simulink model "sam"  (R2016b)
settings: Solver=VariableStepAuto  StartTime=0.0  StopTime=10  FixedStep=0.00001
values from neighbouring files (symbols this model uses):
  J = 0.0025    [momentFun.m]
  K = Kf*R/Km+Ke    (= 4.8)    [momentFun.m]
  Kd = Kn(3)    [momentFun.m]
  Ki = Kn(2)    [momentFun.m]
  Km = 4.8    [momentFun.m]
  Kp = Kn(1)    [momentFun.m]
  maxV = 6.8    [momentFun.m]
  R = 5.2    [momentFun.m]
libraries: simulink x1
settings Model: Creator=texnoman  LastModifiedBy=texnoman
settings SolverCC: MaxConsecutiveMinStep=auto  ZeroCrossControl=DisableAll

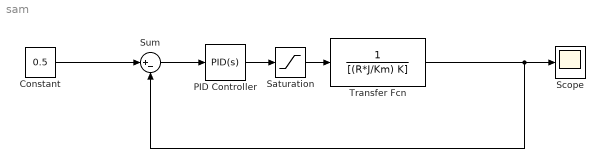
== system sam ==
  Constant : Constant  Value=0.5
  PID Controller : simulink/Continuous/PID Controller  Controller=PID  TimeDomain=Continuous-time  SampleTime=-1  IntegratorMethod=Forward Euler  FilterMethod=Forward Euler  Form=Parallel  UseFilter=on  ControllerParametersSource=internal  P=Kp  I=Ki  D=Kd  N=100  InitialConditionSource=internal  InitialConditionForIntegrator=0  InitialConditionForFilter=0  ExternalReset=none  LimitOutput=off  UpperSaturationLimit=inf  LowerSaturationLimit=-inf  LinearizeAsGain=on  AntiWindupMode=none  Kb=1  TrackingMode=off  Kt=1  PParamMin=[]  PParamMax=[]  IParamMin=[]  IParamMax=[]  DParamMin=[]  DParamMax=[]  NParamMin=[]  NParamMax=[]  KbParamMin=[]  KbParamMax=[]  KtParamMin=[]  KtParamMax=[]  POutMin=[]  POutMax=[]  IOutMin=[]  IOutMax=[]  DOutMin=[]  DOutMax=[]  NOutMin=[]  NOutMax=[]  KbOutMin=[]  KbOutMax=[]  KtOutMin=[]  KtOutMax=[]  IntegratorOutMin=[]  IntegratorOutMax=[]  FilterOutMin=[]  FilterOutMax=[]  SumOutMin=[]  SumOutMax=[]  SumI1OutMin=[]  SumI1OutMax=[]  SumI2OutMin=[]  SumI2OutMax=[]  SumI3OutMin=[]  SumI3OutMax=[]  SumDOutMin=[]  SumDOutMax=[]  SaturationOutMin=[]  SaturationOutMax=[]  IntegratorContinuousStateAttributes=''  IntegratorStateMustResolveToSignalObject=off  IntegratorRTWStateStorageClass=Auto  FilterContinuousStateAttributes=''  FilterStateMustResolveToSignalObject=off  FilterRTWStateStorageClass=Auto  DifferentiatorICPrevScaledInput=0  DifferentiatorOutMin=[]  DifferentiatorOutMax=[]
  Saturation : Saturate  UpperLimit=maxV  LowerLimit=-maxV
  Scope : Scope
  Sum : Sum  Inputs=|+-
  Transfer Fcn : TransferFcn  Denominator=[(R*J/Km) K]
  wires:
  PID Controller/1 -> Saturation/1
  Transfer Fcn/1 -> Scope/1, Sum/2
  Sum/1 -> PID Controller/1
  Constant/1 -> Sum/1
  Saturation/1 -> Transfer Fcn/1
